simulink model "Inverter_Trifase_PWM_23"  (R2023b)
settings: Solver=ode23s  StartTime=0.0  StopTime=5
values from neighbouring files (symbols this model uses):
  Lc = 10e-3    (= 0.01)    [data.m]
  Rc = 20    [data.m]
  tau = 0.1    [data.m]
  Tc = 100e-6    (= 0.0001)    [data.m]
undefined symbols (not defined in the file or in its folder): DiscIntNeverNeededParam
libraries: fl_lib x80, nesl_utility x51, slpidlib x3, simulink x1
(part 1 of 2)
settings Model: Creator=Student  LastModifiedBy=francesco.bazzani
settings SolverCC: AlgebraicLoopSolver=TrustRegion
settings DataIOCC: SaveFormat=Array  ReturnWorkspaceOutputs=off
settings DebuggingCC: UnconnectedInputMsg=warning  UnconnectedOutputMsg=warning  UnconnectedLineMsg=warning  ArithmeticOperatorsInVariantConditions=warning
settings ModelReferenceCC: EnableRefExpFcnMdlSchedulingChecks=on
settings SFSimCC: SimUseLocalCustomCode=off  CustomCodeUndefinedFunction=UseInterfaceOnly
settings RTWCC: RTWUseLocalCustomCode=off
settings CodeAppCC: StateflowObjectComments=on
settings SimscapeCC: SimscapeNormalizeSystem=off

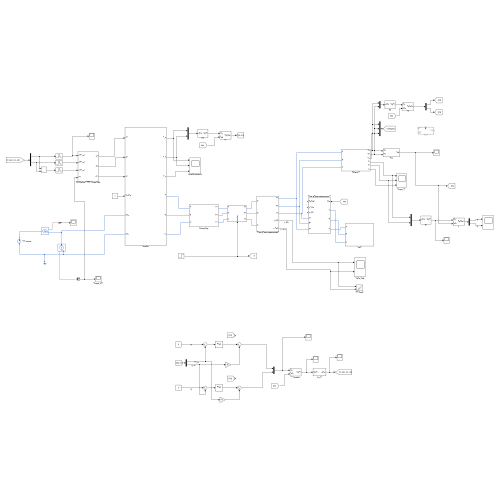
[thumbnail: Simulink's stored preview of the top-level diagram]
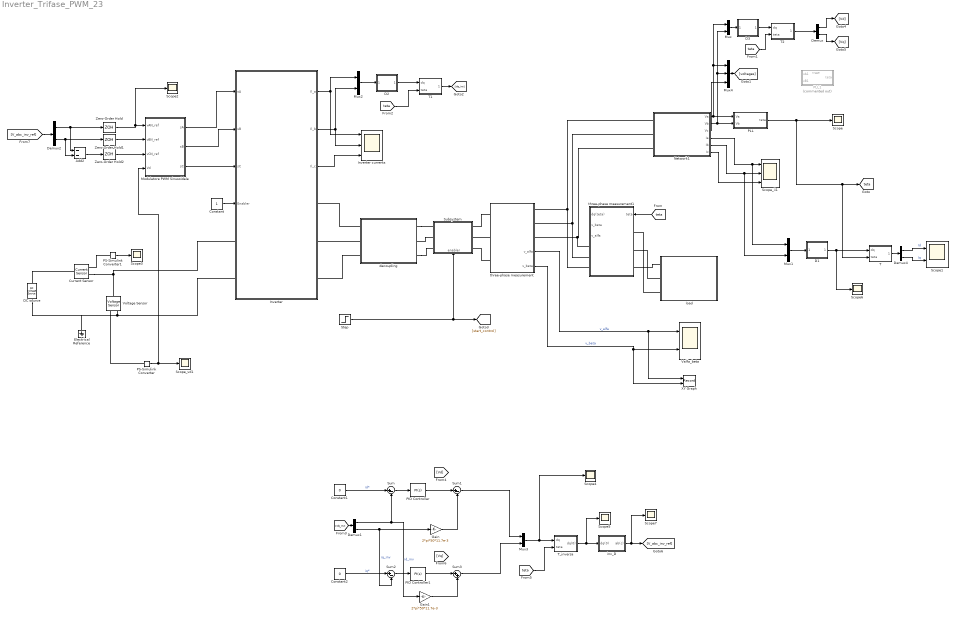
== system Inverter_Trifase_PWM_23 ==
  Add2 : Sum  Inputs=--
  Constant : Constant
  Constant1 : Constant  Value=0
  Constant2 : Constant  Value=0
  Current Sensor : fl_lib/Electrical/Electrical Sensors/Current Sensor
  D1 : Subsystem
  D2 : Subsystem
  D3 : Subsystem
  DC source : fl_lib/Electrical/Electrical Sources/DC Voltage Source  v0=Vd V
  Demux{,1..2,4} (4 alike) : Demux  Outputs=2
  Electrical Reference : fl_lib/Electrical/Electrical Elements/Electrical Reference
  Gain : Gain  Gain=2*pi*50*11.7e-3
  Gain1 : Gain  Gain=2*pi*50*11.7e-3
  Inverter : Subsystem
  Inverter currents : Scope  NumInputPorts=3
  Modulatore PWM Sinusoidale : Subsystem
  Mux{,1..3} (4 alike) : Mux  Inputs=2
  Mux4 : Mux  Inputs=3
  Network1 : Subsystem  mask{E_eff=230, f=50, phi=0}
      mask prompts: f "frequency"; phi "initial_phase"
  PID Controller : slpidlib/PID Controller  Controller=PI  Form=Parallel  TimeDomain=Continuous-time  UseExternalTs=off  SampleTime=-1  IntegratorMethod=Forward Euler  FilterMethod=Forward Euler  ControllerParametersSource=internal  P=Lc/tau  I=Rc/tau  UseKiTs=off  D=0  N=100  UseFilter=on  TunerSelectOption=Transfer Function Based (PID Tuner App)  InitialConditionSource=internal  InitialConditionForIntegrator=0  InitialConditionForFilter=0  DifferentiatorICPrevScaledInput=0  ExternalReset=none  TrackingMode=off  Kt=1  LimitOutput=off  SatLimitsSource=internal  UpperSaturationLimit=inf  LowerSaturationLimit=-inf  LinearizeAsGain=on  AntiWindupMode=none  Kb=1  LimitIntegrator=off  UpperIntegratorSaturationLimit=inf  LowerIntegratorSaturationLimit=-inf  POutMin=[]  POutMax=[]  IOutMin=[]  IOutMax=[]  DOutMin=[]  DOutMax=[]  NOutMin=[]  NOutMax=[]  SumOutMin=[]  SumOutMax=[]  SaturationOutMin=[]  SaturationOutMax=[]  PParamMin=[]  PParamMax=[]  IParamMin=[]  IParamMax=[]  DParamMin=[]  DParamMax=[]  NParamMin=[]  NParamMax=[]  KbParamMin=[]  KbParamMax=[]  KtParamMin=[]  KtParamMax=[]  KbOutMin=[]  KbOutMax=[]  KtOutMin=[]  KtOutMax=[]  IntegratorOutMin=[]  IntegratorOutMax=[]  FilterOutMin=[]  FilterOutMax=[]  SumI1OutMin=[]  SumI1OutMax=[]  SumI2OutMin=[]  SumI2OutMax=[]  SumI3OutMin=[]  SumI3OutMax=[]  SumI4OutMin=[]  SumI4OutMax=[]  SumDOutMin=[]  SumDOutMax=[]  DifferentiatorOutMin=[]  DifferentiatorOutMax=[]  FilterDiffOutCoefMin=[]  FilterDiffOutCoefMax=[]  ReciprocalOutMin=[]  ReciprocalOutMax=[]  SumDenOutMin=[]  SumDenOutMax=[]  SumNumOutMin=[]  SumNumOutMax=[]  DivideOutMin=[]  DivideOutMax=[]  UdiffTsProdOutMin=[]  UdiffTsProdOutMax=[]  NTsProdOutMin=[]  NTsProdOutMax=[]  UintegralTsProdOutMin=[]  UintegralTsProdOutMax=[]  UngainTsProdOutMin=[]  UngainTsProdOutMax=[]  ClampingZeroOutDataTypeStr=Inherit: Inherit via back propagation  ClampingZeroOutMin=[]  ClampingZeroOutMax=[]  FilterDenConstantOutDataTypeStr=Inherit: Inherit via back propagation  FilterDenConstantOutMin=[]  FilterDenConstantOutMax=[]  PCopyOutDataTypeStr=Inherit: Inherit via back propagation  PCopyOutMin=[]  PCopyOutMax=[]  NCopyOutDataTypeStr=Inherit: Inherit via back propagation  NCopyOutMin=[]  NCopyOutMax=[]  IntegratorContinuousStateAttributes=''  IntegratorStateMustResolveToSignalObject=off  IntegratorRTWStateStorageClass=Auto  FilterContinuousStateAttributes=''  FilterStateMustResolveToSignalObject=off  FilterRTWStateStorageClass=Auto  ParallelPVariant=InternalParameters  IdealPVariant=Disabled  IVariant=InternalParameters  DVariant=Disabled  IntegratorVariant=Continuous  SatVariant=Disabled  AWVariant=Passthrough  PCopyVariant=Disabled  TRVariant=Disabled  FdbkBlocksVariant=Forward  IdealPFdbkVariant=Disabled  SatFdbkVariant=Disabled  DerivativeFilterVariant=Disabled  NVariant=Disabled  NCopyVariant=Disabled_SignalSpec  FilterICVariant=Disabled  IntegratorICVariant=InternalICs  ExternalResetVariant=Disabled  TRSumVariant=Passthrough  SumFdbkVariant=Disabled  SumVariant=Sum_PI  TsampFilterVariant=InternalTs  TsampNgainVariant=Passthrough  TsampIntegralVariant=Disabled_SignalSpec  ExternalSaturationOutDataTypeStr=Inherit: Same as second input
  PID Controller1 : slpidlib/PID Controller  Controller=PI  Form=Parallel  TimeDomain=Continuous-time  UseExternalTs=off  SampleTime=-1  IntegratorMethod=Forward Euler  FilterMethod=Forward Euler  ControllerParametersSource=internal  P=Lc/tau  I=Rc/tau  UseKiTs=off  D=0  N=100  UseFilter=on  TunerSelectOption=Transfer Function Based (PID Tuner App)  InitialConditionSource=internal  InitialConditionForIntegrator=0  InitialConditionForFilter=0  DifferentiatorICPrevScaledInput=0  ExternalReset=none  TrackingMode=off  Kt=1  LimitOutput=off  SatLimitsSource=internal  UpperSaturationLimit=inf  LowerSaturationLimit=-inf  LinearizeAsGain=on  AntiWindupMode=none  Kb=1  LimitIntegrator=off  UpperIntegratorSaturationLimit=inf  LowerIntegratorSaturationLimit=-inf  POutMin=[]  POutMax=[]  IOutMin=[]  IOutMax=[]  DOutMin=[]  DOutMax=[]  NOutMin=[]  NOutMax=[]  SumOutMin=[]  SumOutMax=[]  SaturationOutMin=[]  SaturationOutMax=[]  PParamMin=[]  PParamMax=[]  IParamMin=[]  IParamMax=[]  DParamMin=[]  DParamMax=[]  NParamMin=[]  NParamMax=[]  KbParamMin=[]  KbParamMax=[]  KtParamMin=[]  KtParamMax=[]  KbOutMin=[]  KbOutMax=[]  KtOutMin=[]  KtOutMax=[]  IntegratorOutMin=[]  IntegratorOutMax=[]  FilterOutMin=[]  FilterOutMax=[]  SumI1OutMin=[]  SumI1OutMax=[]  SumI2OutMin=[]  SumI2OutMax=[]  SumI3OutMin=[]  SumI3OutMax=[]  SumI4OutMin=[]  SumI4OutMax=[]  SumDOutMin=[]  SumDOutMax=[]  DifferentiatorOutMin=[]  DifferentiatorOutMax=[]  FilterDiffOutCoefMin=[]  FilterDiffOutCoefMax=[]  ReciprocalOutMin=[]  ReciprocalOutMax=[]  SumDenOutMin=[]  SumDenOutMax=[]  SumNumOutMin=[]  SumNumOutMax=[]  DivideOutMin=[]  DivideOutMax=[]  UdiffTsProdOutMin=[]  UdiffTsProdOutMax=[]  NTsProdOutMin=[]  NTsProdOutMax=[]  UintegralTsProdOutMin=[]  UintegralTsProdOutMax=[]  UngainTsProdOutMin=[]  UngainTsProdOutMax=[]  ClampingZeroOutDataTypeStr=Inherit: Inherit via back propagation  ClampingZeroOutMin=[]  ClampingZeroOutMax=[]  FilterDenConstantOutDataTypeStr=Inherit: Inherit via back propagation  FilterDenConstantOutMin=[]  FilterDenConstantOutMax=[]  PCopyOutDataTypeStr=Inherit: Inherit via back propagation  PCopyOutMin=[]  PCopyOutMax=[]  NCopyOutDataTypeStr=Inherit: Inherit via back propagation  NCopyOutMin=[]  NCopyOutMax=[]  IntegratorContinuousStateAttributes=''  IntegratorStateMustResolveToSignalObject=off  IntegratorRTWStateStorageClass=Auto  FilterContinuousStateAttributes=''  FilterStateMustResolveToSignalObject=off  FilterRTWStateStorageClass=Auto  ParallelPVariant=InternalParameters  IdealPVariant=Disabled  IVariant=InternalParameters  DVariant=Disabled  IntegratorVariant=Continuous  SatVariant=Disabled  AWVariant=Passthrough  PCopyVariant=Disabled  TRVariant=Disabled  FdbkBlocksVariant=Forward  IdealPFdbkVariant=Disabled  SatFdbkVariant=Disabled  DerivativeFilterVariant=Disabled  NVariant=Disabled  NCopyVariant=Disabled_SignalSpec  FilterICVariant=Disabled  IntegratorICVariant=InternalICs  ExternalResetVariant=Disabled  TRSumVariant=Passthrough  SumFdbkVariant=Disabled  SumVariant=Sum_PI  TsampFilterVariant=InternalTs  TsampNgainVariant=Passthrough  TsampIntegralVariant=Disabled_SignalSpec  ExternalSaturationOutDataTypeStr=Inherit: Same as second input
  PLL : Subsystem
  PLL1 : Subsystem  Commented=on  mask{ki=500, kp=0.5, f=50}
      mask prompts: f "frequency"
  PS-Simulink Converter : nesl_utility/PS-Simulink Converter  PhysicalDomain=network_engine_domain  SubClassName=ps_output  LeftPortType=input  RightPortType=output  PseudoPeriodic=off  Frequencies=[]  VectorFormat=inherit  Unit=inherit  AffineConversion=off
  PS-Simulink Converter1 : nesl_utility/PS-Simulink Converter  PhysicalDomain=network_engine_domain  SubClassName=ps_output  LeftPortType=input  RightPortType=output  PseudoPeriodic=off  Frequencies=[]  VectorFormat=inherit  Unit=inherit  AffineConversion=off
  Scope{,2..7} (7 alike) : Scope
  Scope1 : Scope  NumInputPorts=2
  Scope_ii1 : Scope  NumInputPorts=3
  Scope_vd1 : Scope
  Step : Step  Time=0  SampleTime=0
  Subsystem : Subsystem
      settings: PortSchema="{\"entries\":[{\"content\":{\"sides\":[{\"content\":{\"connectorIds\":[\"LConn1\",\"LConn2\",\"LConn3\"]},\"type\":\"ConnectorPlacement.EquallySpacedRectSide\",\"uuid\":\"d73297a6-9a93-4c36-8ae1-6d58b261bf06\"},{\"content\":{\"connectorIds\":[\"RConn1\",\"RConn2\",\"RConn3\"],\"side\":\"RIGHT\"},\"type\":\"ConnectorPlacement.EquallySpacedRectSide\",\"uuid\":\"6086bef5-aae9-4392-b869-029ceeb45d41\"},{\"content\":{\"side\":\"TOP\"},\"type\":\"ConnectorPlacement.EquallySpacedRectSide\",\"uuid\":\"d2ebd610-1944-41f8-9294-13f98c946317\"},{\"content\":{\"connectorIds\":[\"In1\"],\"side\":\"BOTTOM\"},\"type\":\"ConnectorPlacement.EquallySpacedRectSide\",\"uuid\":\"967f94e7-9c23-48ce-995b-e38326ca9967\"}]},\"type\":\"ConnectorPlacement.EquallySpacedConnector\",\"uuid\":\"e9d282ac-9c88-4679-adaa-ae858ea7366f\"}],\"packageUris\":[\"http://schema.mathworks.com/mf0/Connector/R2020b\"],\"version\":\"1.0\"}"
  Sum : Sum  Inputs=|+-
  Sum1 : Sum  Inputs=|+-
  Sum2 : Sum  Inputs=|+-
  Sum3 : Sum  Inputs=|++
  T : Subsystem
  T1 : Subsystem
  T2 : Subsystem
  T_inversa : Subsystem
  Valfa_beta : Scope  NumInputPorts=2
  Voltage Sensor : fl_lib/Electrical/Electrical Sensors/Voltage Sensor
  XY Graph : Record  FileSettingsInternal="{\"entries\":[{\"content\":{\"excelSettings\":{\"content\":{},\"type\":\"Streamout.ExcelSettings\"}},\"type\":\"Streamout.FileSettingStorage\",\"uuid\":\"\"}],\"packageUris\":[\"http:\\/\\/schema.mathworks.com\\/mf0\\/streamout_blocks\\/R2020a\"],\"version\":\"1.0\"}"  Layout=[1 1]  SignalsInternal="{\"entries\":[{\"content\":{\"signals\":[{\"content\":{\"blockPath\":[],\"dimensions\":[1],\"domain\":\"\",\"lineColor\":\"#77ac30\",\"lineWidth\":2,\"port\":1,\"signalID\":1,\"signalName\":\"v_alfa\"},\"type\":\"RecordBlkView.Signal\",\"uuid\":\"\"},{\"content\":{\"blockPath\":[],\"dimensions\":[1],\"domain\":\"\",\"lineColor\":\"#4dbeee\",\"lineWidth\":2,\"port\":2,\"signalID\":2,\"signalName\":\"v_beta\"},\"type\":\"RecordBlkView.Signal\",\"uuid\":\"\"}]},\"type\":\"RecordBlkView.InputSignals\",\"uuid\":\"\"}],\"packageUris\":[\"http:\\/\\/schema.mathworks.com\\/mf0\\/streamout_blocks\\/R2020a\"],\"version\":\"1.0\"}"  VisualizationBindings="{\"xyplotplugin\":{\"info\":[{\"series\":[],\"subplotID\":1}]}}"  CompatibilityTag=XY
  Zero-Order Hold : ZeroOrderHold  SampleTime=Tc
  Zero-Order Hold1 : ZeroOrderHold  SampleTime=Tc
  Zero-Order Hold2 : ZeroOrderHold  SampleTime=Tc
  decoupling : Subsystem  mask{Rc=1e-9, Lc=9e-3}
      mask prompts: Rc "Resistor"; Lc "Inductance"
  inv_D : Subsystem
  load : Subsystem  mask{Rc=Rc, Lc=Lc, Cc=0.1e-9}
      mask prompts: Rc "Resistor"; Lc "Inductance"; Cc "Capacitance"
  three-phase measurement : Subsystem
      settings: PortSchema="{\"entries\":[{\"content\":{\"sides\":[{\"content\":{\"connectorIds\":[\"LConn1\",\"LConn2\",\"LConn3\"]},\"type\":\"ConnectorPlacement.EquallySpacedRectSide\",\"uuid\":\"32d21379-5403-4c81-86bb-b48365f60f54\"},{\"content\":{\"connectorIds\":[\"RConn1\",\"RConn2\",\"RConn3\",\"Out1\",\"Out2\"],\"side\":\"RIGHT\"},\"type\":\"ConnectorPlacement.EquallySpacedRectSide\",\"uuid\":\"24ab37a8-a81a-4881-af76-f78c15280390\"},{\"content\":{\"side\":\"TOP\"},\"type\":\"ConnectorPlacement.EquallySpacedRectSide\",\"uuid\":\"2c2ce5b3-2749-4524-8cf7-f3135c13c1a5\"}]},\"type\":\"ConnectorPlacement.EquallySpacedConnector\",\"uuid\":\"48562a3f-ee3b-41f1-a0b2-9ed72f3d9b82\"}],\"packageUris\":[\"http://schema.mathworks.com/mf0/Connector/R2020b\"],\"version\":\"1.0\"}"
  three-phase measurement1 : Subsystem
      settings: PortSchema="{\"entries\":[{\"content\":{\"sides\":[{\"content\":{\"connectorIds\":[\"LConn1\",\"LConn2\",\"LConn3\",\"In1\"]},\"type\":\"ConnectorPlacement.EquallySpacedRectSide\",\"uuid\":\"32d21379-5403-4c81-86bb-b48365f60f54\"},{\"content\":{\"connectorIds\":[\"RConn1\",\"RConn2\",\"RConn3\",\"Out1\",\"Out2\",\"Out3\"],\"side\":\"RIGHT\"},\"type\":\"ConnectorPlacement.EquallySpacedRectSide\",\"uuid\":\"24ab37a8-a81a-4881-af76-f78c15280390\"},{\"content\":{\"side\":\"TOP\"},\"type\":\"ConnectorPlacement.EquallySpacedRectSide\",\"uuid\":\"2c2ce5b3-2749-4524-8cf7-f3135c13c1a5\"}]},\"type\":\"ConnectorPlacement.EquallySpacedConnector\",\"uuid\":\"48562a3f-ee3b-41f1-a0b2-9ed72f3d9b82\"}],\"packageUris\":[\"http://schema.mathworks.com/mf0/Connector/R2020b\"],\"version\":\"1.0\"}"
  tag scope: teta=global
  wires:
  Zero-Order Hold/1 -> Scope2/1, Modulatore PWM Sinusoidale/1(vAN_ref)
  Zero-Order Hold1/1 -> Modulatore PWM Sinusoidale/2(vBN_ref)
  Zero-Order Hold2/1 -> Modulatore PWM Sinusoidale/3(vCN_ref)
  PS-Simulink Converter/1 -> Modulatore PWM Sinusoidale/4(Vd), Scope_vd1/1
  Modulatore PWM Sinusoidale/2(sB) -> Inverter/2(sB)
  Modulatore PWM Sinusoidale/3(sC) -> Inverter/3(sC)
  Modulatore PWM Sinusoidale/1(sA) -> Inverter/1(sA)
  three-phase measurement/1(v_alfa) -> Valfa_beta/1, XY Graph/1  "v_alfa"
  three-phase measurement/2(v_beta) -> XY Graph/2, Valfa_beta/2  "v_beta"
  PLL/1(teta) -> T/2(teta), [teta], Scope/1
  Network1/1(Va) -> Mux/1, Mux4/1, PLL/1(Va)
  Network1/2(Vb) -> Mux/2, Mux4/2, PLL/2(Vb)
  Network1/6(Ic) -> Scope_ii1/3
  Network1/5(Ib) -> Mux1/2, Scope_ii1/2
  Mux1/1 -> D1/1(ab(c))
  Network1/4(Ia) -> Mux1/1, Scope_ii1/1
  PS-Simulink Converter1/1 -> Scope3/1
  Inverter/1(Il_a) -> Inverter currents/1, Mux2/1
  Inverter/2(Il_b) -> Inverter currents/2, Mux2/2
  Inverter/3(Il_c) -> Inverter currents/3
  Mux2/1 -> D2/1(ab(c))
  D2/1(dq(0)) -> T1/1(dq)
  [teta] -> T1/2(teta)
  T1/1(dq(teta)) -> [idq_inv]
  D1/1(dq(0)) -> Scope6/1, T/1(dq)
  T/1(dq(teta)) -> Demux4/1
  Demux4/1 -> Scope1/1  "Id"
  Demux4/2 -> Scope1/2  "Iq"
  Network1/3(Vc) -> Mux4/3
  Mux4/1 -> [voltages]
  Constant/1 -> Inverter/4(Enabler)
  Step/1 -> Subsystem/1(enabler), [start_control]
  [teta] -> three-phase measurement1/1(teta)
  Mux/1 -> D3/1(ab(c))
  D3/1(dq(0)) -> T2/1(dq)
  [teta] -> T2/2(teta)
  T2/1(dq(teta)) -> Demux/1
  Demux/1 -> [Vd]
  Demux/2 -> [Vq]
  Constant1/1 -> Sum/1  "id*"
  [idq_inv] -> Demux1/1
  Demux1/1 -> Gain1/1, Sum/2  "id_inv"
  Sum/1 -> PID Controller/1
  Demux1/2 -> Sum2/2, Gain/1  "iq_inv"
  Gain/1 -> Sum1/2
  PID Controller/1 -> Sum1/1
  PID Controller1/1 -> Sum3/1
  Gain1/1 -> Sum3/2
  Sum2/1 -> PID Controller1/1
  Constant2/1 -> Sum2/1  "iq*"
  Sum1/1 -> Mux3/1
  Sum3/1 -> Mux3/2
  Mux3/1 -> Scope4/1, T_inversa/1(dq)
  [teta] -> T_inversa/2(teta)
  T_inversa/1(dq(0)) -> Scope5/1, inv_D/1(dq(0))
  inv_D/1(ab(c)) -> Scope7/1, [V_abc_inv_ref]
  [V_abc_inv_ref] -> Demux2/1
  Demux2/1 -> Add2/1, Zero-Order Hold/1
  Demux2/2 -> Add2/2, Zero-Order Hold1/1
  Add2/1 -> Zero-Order Hold2/1
  connections:
  Inverter/LConn1 -- Voltage Sensor/LConn1 -- Current Sensor/RConn2
  Voltage Sensor/RConn2 -- DC source/RConn1 -- Electrical Reference/LConn1 -- Inverter/LConn2
  PS-Simulink Converter/LConn1 -- Voltage Sensor/RConn1
  Network1/LConn1 -- three-phase measurement1/RConn1 -- three-phase measurement/RConn1
  Network1/LConn2 -- three-phase measurement1/RConn2 -- three-phase measurement/RConn2
  Network1/LConn3 -- three-phase measurement1/RConn3 -- three-phase measurement/RConn3
  Current Sensor/LConn1 -- DC source/LConn1
  PS-Simulink Converter1/LConn1 -- Current Sensor/RConn1
  three-phase measurement/LConn1 -- Subsystem/LConn1
  three-phase measurement/LConn2 -- Subsystem/LConn2
  three-phase measurement/LConn3 -- Subsystem/LConn3
  decoupling/LConn1 -- Inverter/RConn1
  decoupling/LConn2 -- Inverter/RConn2
  decoupling/LConn3 -- Inverter/RConn3
  Subsystem/RConn2 -- decoupling/RConn2
  decoupling/RConn3 -- Subsystem/RConn3
  decoupling/RConn1 -- Subsystem/RConn1
  load/LConn1 -- three-phase measurement1/LConn1
  load/LConn2 -- three-phase measurement1/LConn2
  load/LConn3 -- three-phase measurement1/LConn3

== system Inverter_Trifase_PWM_23/D1 ==
  ab(c) : Inport
  Gain : Gain  Gain=[1 0; 1/sqrt(3) 2/sqrt(3)]  Multiplication=Matrix(K*u)
  dq(0) : Outport
  wires:
  ab(c)/1 -> Gain/1
  Gain/1 -> dq(0)/1

== system Inverter_Trifase_PWM_23/D2 ==
  ab(c) : Inport
  Gain : Gain  Gain=[1 0; 1/sqrt(3) 2/sqrt(3)]  Multiplication=Matrix(K*u)
  dq(0) : Outport
  wires:
  Gain/1 -> dq(0)/1
  ab(c)/1 -> Gain/1

== system Inverter_Trifase_PWM_23/D3 ==
  ab(c) : Inport
  Gain : Gain  Gain=[1 0; 1/sqrt(3) 2/sqrt(3)]  Multiplication=Matrix(K*u)
  dq(0) : Outport
  wires:
  Gain/1 -> dq(0)/1
  ab(c)/1 -> Gain/1

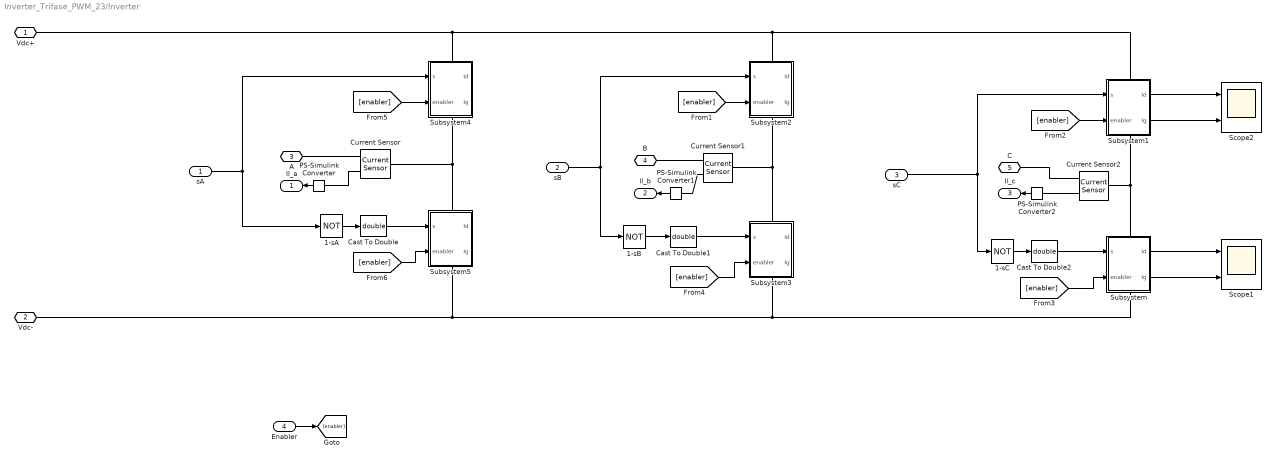
== system Inverter_Trifase_PWM_23/Inverter ==
  sA : Inport
  sB : Inport  Port=2
  sC : Inport  Port=3
  Enabler : Inport  Port=4
  1-sA : Logic  Operator=NOT  AllPortsSameDT=off  OutDataTypeStr=boolean
  1-sB : Logic  Operator=NOT  AllPortsSameDT=off  OutDataTypeStr=boolean
  1-sC : Logic  Operator=NOT  AllPortsSameDT=off  OutDataTypeStr=boolean
  Cast To Double : DataTypeConversion  OutDataTypeStr=double  SaturateOnIntegerOverflow=off  RndMeth=Floor
  Cast To Double1 : DataTypeConversion  OutDataTypeStr=double  SaturateOnIntegerOverflow=off  RndMeth=Floor
  Cast To Double2 : DataTypeConversion  OutDataTypeStr=double  SaturateOnIntegerOverflow=off  RndMeth=Floor
  Current Sensor : fl_lib/Electrical/Electrical Sensors/Current Sensor
  Current Sensor1 : fl_lib/Electrical/Electrical Sensors/Current Sensor
  Current Sensor2 : fl_lib/Electrical/Electrical Sensors/Current Sensor
  PS-Simulink Converter : nesl_utility/PS-Simulink Converter  PhysicalDomain=network_engine_domain  SubClassName=ps_output  LeftPortType=input  RightPortType=output  PseudoPeriodic=off  Frequencies=[]  VectorFormat=inherit  Unit=inherit  AffineConversion=off
  PS-Simulink Converter1 : nesl_utility/PS-Simulink Converter  PhysicalDomain=network_engine_domain  SubClassName=ps_output  LeftPortType=input  RightPortType=output  PseudoPeriodic=off  Frequencies=[]  VectorFormat=inherit  Unit=inherit  AffineConversion=off
  PS-Simulink Converter2 : nesl_utility/PS-Simulink Converter  PhysicalDomain=network_engine_domain  SubClassName=ps_output  LeftPortType=input  RightPortType=output  PseudoPeriodic=off  Frequencies=[]  VectorFormat=inherit  Unit=inherit  AffineConversion=off
  Scope1 : Scope  NumInputPorts=2
  Scope2 : Scope  NumInputPorts=2
  Subsystem : Subsystem
      settings: PortSchema="{\"entries\":[{\"content\":{\"sides\":[{\"content\":{\"connectorIds\":[\"In1\",\"In2\"]},\"type\":\"ConnectorPlacement.EquallySpacedRectSide\",\"uuid\":\"4e5f692d-a64c-483a-ac5e-cd512d23b242\"},{\"content\":{\"connectorIds\":[\"Out1\",\"Out2\"],\"side\":\"RIGHT\"},\"type\":\"ConnectorPlacement.EquallySpacedRectSide\",\"uuid\":\"e12fe3d4-c0cd-4a3e-9242-ad46fbec7d56\"},{\"content\":{\"connectorIds\":[\"LConn1\"],\"side\":\"TOP\"},\"type\":\"ConnectorPlacement.EquallySpacedRectSide\",\"uuid\":\"d4554ec2-8758-4e5e-9cf9-0240d1caee6b\"},{\"content\":{\"connectorIds\":[\"RConn1\"],\"side\":\"BOTTOM\"},\"type\":\"ConnectorPlacement.EquallySpacedRectSide\",\"uuid\":\"09a039c2-054f-4084-afc4-ab4cf2e2d665\"}]},\"type\":\"ConnectorPlacement.EquallySpacedConnector\",\"uuid\":\"56f78543-d3be-4c9c-bdd6-bf2d059f1aee\"}],\"packageUris\":[\"http://schema.mathworks.com/mf0/Connector/R2020b\"],\"version\":\"1.0\"}"
  Subsystem1 : Subsystem
      settings: PortSchema="{\"entries\":[{\"content\":{\"sides\":[{\"content\":{\"connectorIds\":[\"In1\",\"In2\"]},\"type\":\"ConnectorPlacement.EquallySpacedRectSide\",\"uuid\":\"4e5f692d-a64c-483a-ac5e-cd512d23b242\"},{\"content\":{\"connectorIds\":[\"Out1\",\"Out2\"],\"side\":\"RIGHT\"},\"type\":\"ConnectorPlacement.EquallySpacedRectSide\",\"uuid\":\"e12fe3d4-c0cd-4a3e-9242-ad46fbec7d56\"},{\"content\":{\"connectorIds\":[\"LConn1\"],\"side\":\"TOP\"},\"type\":\"ConnectorPlacement.EquallySpacedRectSide\",\"uuid\":\"d4554ec2-8758-4e5e-9cf9-0240d1caee6b\"},{\"content\":{\"connectorIds\":[\"RConn1\"],\"side\":\"BOTTOM\"},\"type\":\"ConnectorPlacement.EquallySpacedRectSide\",\"uuid\":\"09a039c2-054f-4084-afc4-ab4cf2e2d665\"}]},\"type\":\"ConnectorPlacement.EquallySpacedConnector\",\"uuid\":\"56f78543-d3be-4c9c-bdd6-bf2d059f1aee\"}],\"packageUris\":[\"http://schema.mathworks.com/mf0/Connector/R2020b\"],\"version\":\"1.0\"}"
  Subsystem2 : Subsystem
      settings: PortSchema="{\"entries\":[{\"content\":{\"sides\":[{\"content\":{\"connectorIds\":[\"In1\",\"In2\"]},\"type\":\"ConnectorPlacement.EquallySpacedRectSide\",\"uuid\":\"4e5f692d-a64c-483a-ac5e-cd512d23b242\"},{\"content\":{\"connectorIds\":[\"Out1\",\"Out2\"],\"side\":\"RIGHT\"},\"type\":\"ConnectorPlacement.EquallySpacedRectSide\",\"uuid\":\"e12fe3d4-c0cd-4a3e-9242-ad46fbec7d56\"},{\"content\":{\"connectorIds\":[\"LConn1\"],\"side\":\"TOP\"},\"type\":\"ConnectorPlacement.EquallySpacedRectSide\",\"uuid\":\"d4554ec2-8758-4e5e-9cf9-0240d1caee6b\"},{\"content\":{\"connectorIds\":[\"RConn1\"],\"side\":\"BOTTOM\"},\"type\":\"ConnectorPlacement.EquallySpacedRectSide\",\"uuid\":\"09a039c2-054f-4084-afc4-ab4cf2e2d665\"}]},\"type\":\"ConnectorPlacement.EquallySpacedConnector\",\"uuid\":\"56f78543-d3be-4c9c-bdd6-bf2d059f1aee\"}],\"packageUris\":[\"http://schema.mathworks.com/mf0/Connector/R2020b\"],\"version\":\"1.0\"}"
  Subsystem3 : Subsystem
      settings: PortSchema="{\"entries\":[{\"content\":{\"sides\":[{\"content\":{\"connectorIds\":[\"In1\",\"In2\"]},\"type\":\"ConnectorPlacement.EquallySpacedRectSide\",\"uuid\":\"4e5f692d-a64c-483a-ac5e-cd512d23b242\"},{\"content\":{\"connectorIds\":[\"Out1\",\"Out2\"],\"side\":\"RIGHT\"},\"type\":\"ConnectorPlacement.EquallySpacedRectSide\",\"uuid\":\"e12fe3d4-c0cd-4a3e-9242-ad46fbec7d56\"},{\"content\":{\"connectorIds\":[\"LConn1\"],\"side\":\"TOP\"},\"type\":\"ConnectorPlacement.EquallySpacedRectSide\",\"uuid\":\"d4554ec2-8758-4e5e-9cf9-0240d1caee6b\"},{\"content\":{\"connectorIds\":[\"RConn1\"],\"side\":\"BOTTOM\"},\"type\":\"ConnectorPlacement.EquallySpacedRectSide\",\"uuid\":\"09a039c2-054f-4084-afc4-ab4cf2e2d665\"}]},\"type\":\"ConnectorPlacement.EquallySpacedConnector\",\"uuid\":\"56f78543-d3be-4c9c-bdd6-bf2d059f1aee\"}],\"packageUris\":[\"http://schema.mathworks.com/mf0/Connector/R2020b\"],\"version\":\"1.0\"}"
  Subsystem4 : Subsystem
      settings: PortSchema="{\"entries\":[{\"content\":{\"sides\":[{\"content\":{\"connectorIds\":[\"In1\",\"In2\"]},\"type\":\"ConnectorPlacement.EquallySpacedRectSide\",\"uuid\":\"4e5f692d-a64c-483a-ac5e-cd512d23b242\"},{\"content\":{\"connectorIds\":[\"Out1\",\"Out2\"],\"side\":\"RIGHT\"},\"type\":\"ConnectorPlacement.EquallySpacedRectSide\",\"uuid\":\"e12fe3d4-c0cd-4a3e-9242-ad46fbec7d56\"},{\"content\":{\"connectorIds\":[\"LConn1\"],\"side\":\"TOP\"},\"type\":\"ConnectorPlacement.EquallySpacedRectSide\",\"uuid\":\"d4554ec2-8758-4e5e-9cf9-0240d1caee6b\"},{\"content\":{\"connectorIds\":[\"RConn1\"],\"side\":\"BOTTOM\"},\"type\":\"ConnectorPlacement.EquallySpacedRectSide\",\"uuid\":\"09a039c2-054f-4084-afc4-ab4cf2e2d665\"}]},\"type\":\"ConnectorPlacement.EquallySpacedConnector\",\"uuid\":\"56f78543-d3be-4c9c-bdd6-bf2d059f1aee\"}],\"packageUris\":[\"http://schema.mathworks.com/mf0/Connector/R2020b\"],\"version\":\"1.0\"}"
  Subsystem5 : Subsystem
      settings: PortSchema="{\"entries\":[{\"content\":{\"sides\":[{\"content\":{\"connectorIds\":[\"In1\",\"In2\"]},\"type\":\"ConnectorPlacement.EquallySpacedRectSide\",\"uuid\":\"4e5f692d-a64c-483a-ac5e-cd512d23b242\"},{\"content\":{\"connectorIds\":[\"Out1\",\"Out2\"],\"side\":\"RIGHT\"},\"type\":\"ConnectorPlacement.EquallySpacedRectSide\",\"uuid\":\"e12fe3d4-c0cd-4a3e-9242-ad46fbec7d56\"},{\"content\":{\"connectorIds\":[\"LConn1\"],\"side\":\"TOP\"},\"type\":\"ConnectorPlacement.EquallySpacedRectSide\",\"uuid\":\"d4554ec2-8758-4e5e-9cf9-0240d1caee6b\"},{\"content\":{\"connectorIds\":[\"RConn1\"],\"side\":\"BOTTOM\"},\"type\":\"ConnectorPlacement.EquallySpacedRectSide\",\"uuid\":\"09a039c2-054f-4084-afc4-ab4cf2e2d665\"}]},\"type\":\"ConnectorPlacement.EquallySpacedConnector\",\"uuid\":\"56f78543-d3be-4c9c-bdd6-bf2d059f1aee\"}],\"packageUris\":[\"http://schema.mathworks.com/mf0/Connector/R2020b\"],\"version\":\"1.0\"}"
  Vdc+ : PMIOPort  Side=Left
  Vdc- : PMIOPort  Port=2  Side=Left
  A : PMIOPort  Port=3  Side=Right
  B : PMIOPort  Port=4  Side=Right
  C : PMIOPort  Port=5  Side=Right
  Il_a : Outport
  Il_b : Outport  Port=2
  Il_c : Outport  Port=3
  wires:
  1-sA/1 -> Cast To Double/1
  1-sC/1 -> Cast To Double2/1
  1-sB/1 -> Cast To Double1/1
  Cast To Double1/1 -> Subsystem3/1(s)
  Enabler/1 -> [enabler]
  sA/1 -> 1-sA/1, Subsystem4/1(s)
  sB/1 -> 1-sB/1, Subsystem2/1(s)
  sC/1 -> 1-sC/1, Subsystem1/1(s)
  PS-Simulink Converter/1 -> Il_a/1
  PS-Simulink Converter1/1 -> Il_b/1
  PS-Simulink Converter2/1 -> Il_c/1
  Cast To Double2/1 -> Subsystem/1(s)
  [enabler] -> Subsystem/2(enabler)
  [enabler] -> Subsystem1/2(enabler)
  Subsystem1/1(Id) -> Scope2/1
  Subsystem1/2(Ig) -> Scope2/2
  Subsystem/1(Id) -> Scope1/1
  Subsystem/2(Ig) -> Scope1/2
  [enabler] -> Subsystem2/2(enabler)
  [enabler] -> Subsystem3/2(enabler)
  Cast To Double/1 -> Subsystem5/1(s)
  [enabler] -> Subsystem4/2(enabler)
  [enabler] -> Subsystem5/2(enabler)
  connections:
  Subsystem/LConn1 -- Subsystem1/RConn1 -- Current Sensor2/LConn1
  Subsystem1/LConn1 -- Subsystem2/LConn1 -- Vdc+/RConn1 -- Subsystem4/LConn1
  A/RConn1 -- Current Sensor/RConn2
  Current Sensor/RConn1 -- PS-Simulink Converter/LConn1
  Current Sensor1/RConn2 -- B/RConn1
  PS-Simulink Converter1/LConn1 -- Current Sensor1/RConn1
  Current Sensor2/RConn2 -- C/RConn1
  PS-Simulink Converter2/LConn1 -- Current Sensor2/RConn1
  Subsystem3/RConn1 -- Subsystem5/RConn1 -- Vdc-/RConn1 -- Subsystem/RConn1
  Subsystem3/LConn1 -- Current Sensor1/LConn1 -- Subsystem2/RConn1
  Subsystem5/LConn1 -- Current Sensor/LConn1 -- Subsystem4/RConn1

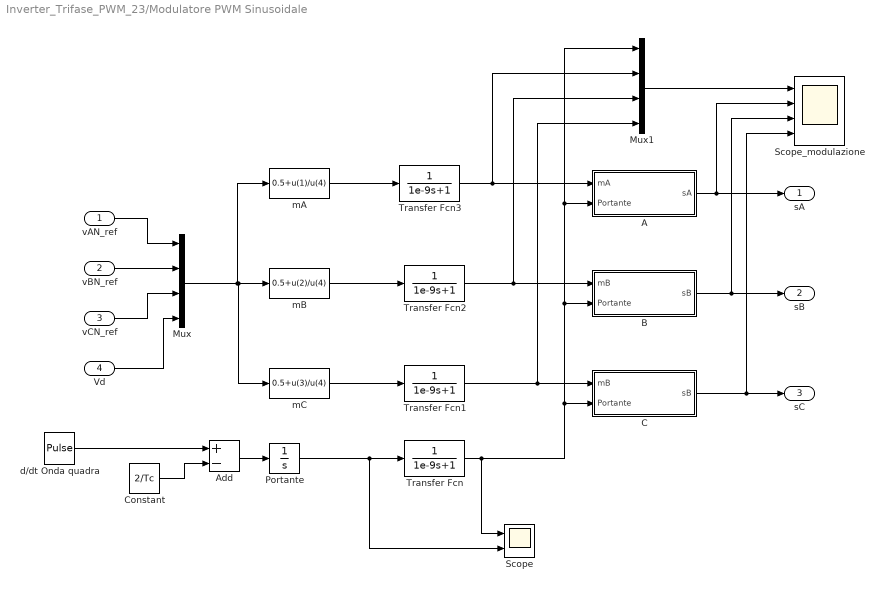
== system Inverter_Trifase_PWM_23/Modulatore PWM Sinusoidale ==
  vAN_ref : Inport
  vBN_ref : Inport  Port=2
  vCN_ref : Inport  Port=3
  Vd : Inport  Port=4
  A : Subsystem
  Add : Sum  Inputs=+-
  B : Subsystem
  C : Subsystem
  Constant : Constant  Value=2/Tc
  Mux : Mux
  Mux1 : Mux
  Portante : Integrator
  Scope : Scope  NumInputPorts=2
  Scope_modulazione : Scope  NumInputPorts=4
  Transfer Fcn{,1..3} (4 alike) : TransferFcn  Denominator=[1e-9 1]
  d/dt Onda quadra : DiscretePulseGenerator  PulseType=Time based  Amplitude=4/Tc  Period=Tc  PulseWidth=50
  mA : Fcn  Expr=0.5+u(1)/u(4)
  mB : Fcn  Expr=0.5+u(2)/u(4)
  mC : Fcn  Expr=0.5+u(3)/u(4)
  sA : Outport  VectorParamsAs1DForOutWhenUnconnected=off
  sB : Outport  Port=2  VectorParamsAs1DForOutWhenUnconnected=off
  sC : Outport  Port=3  VectorParamsAs1DForOutWhenUnconnected=off
  wires:
  d/dt Onda quadra/1 -> Add/1
  Constant/1 -> Add/2
  Add/1 -> Portante/1
  mA/1 -> Transfer Fcn3/1
  Portante/1 -> Scope/2, Transfer Fcn/1
  mB/1 -> Transfer Fcn2/1
  A/1(sA) -> Scope_modulazione/2, sA/1
  B/1(sB) -> Scope_modulazione/3, sB/1
  Mux1/1 -> Scope_modulazione/1
  vAN_ref/1 -> Mux/1
  vBN_ref/1 -> Mux/2
  vCN_ref/1 -> Mux/3
  Vd/1 -> Mux/4
  mC/1 -> Transfer Fcn1/1
  C/1(sB) -> Scope_modulazione/4, sC/1
  Mux/1 -> mA/1, mC/1, mB/1
  Transfer Fcn/1 -> Scope/1, C/2(Portante), B/2(Portante), A/2(Portante), Mux1/1
  Transfer Fcn1/1 -> Mux1/4, C/1(mB)
  Transfer Fcn2/1 -> Mux1/3, B/1(mB)
  Transfer Fcn3/1 -> Mux1/2, A/1(mA)

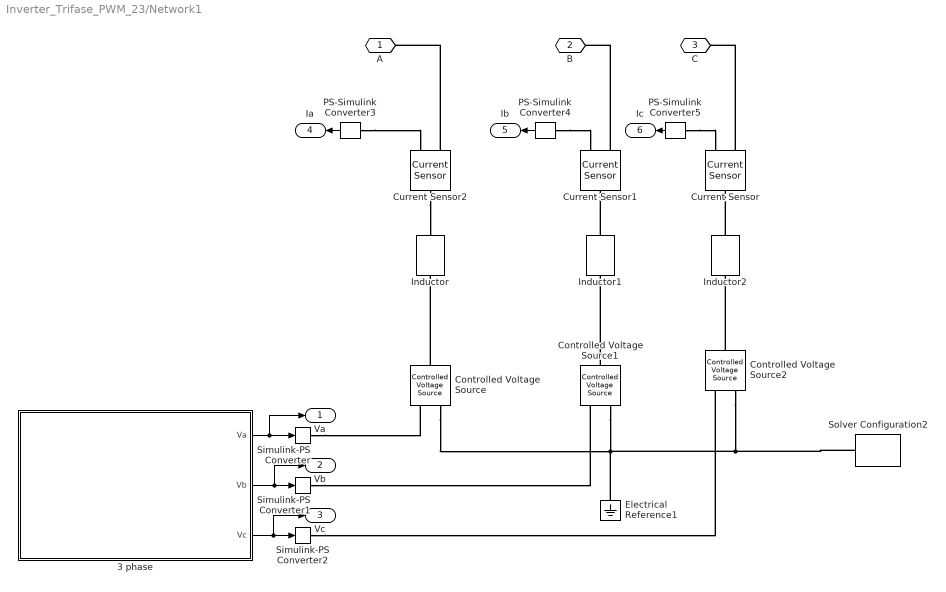
== system Inverter_Trifase_PWM_23/Network1 ==
  3 phase : Subsystem  mask{f=f, Vp=E_eff*sqrt(2)}
      mask prompts: f "Frequency [Hz]"; Vp "Peak value [V]"
  Controlled Voltage Source : fl_lib/Electrical/Electrical Sources/Controlled Voltage Source
  Controlled Voltage Source1 : fl_lib/Electrical/Electrical Sources/Controlled Voltage Source
  Controlled Voltage Source2 : fl_lib/Electrical/Electrical Sources/Controlled Voltage Source
  Current Sensor : fl_lib/Electrical/Electrical Sensors/Current Sensor
  Current Sensor1 : fl_lib/Electrical/Electrical Sensors/Current Sensor
  Current Sensor2 : fl_lib/Electrical/Electrical Sensors/Current Sensor
  Electrical Reference1 : fl_lib/Electrical/Electrical Elements/Electrical Reference
  Inductor : fl_lib/Electrical/Electrical Elements/Inductor  l=2.7e-3 H  r=0 Ohm  g=1e-9 1/Ohm  i_specify=on  i_priority=None  i=0 A  i_nominal_specify=off  i_nominal_value=1  i_nominal_unit=A  v_specify=off  v_priority=None  v=0 V  v_nominal_specify=off  v_nominal_value=1  v_nominal_unit=V  i_L_specify=on  i_L_priority=High  i_L=0 A  i_L_nominal_specify=off  i_L_nominal_value=1  i_L_nominal_unit=A
  Inductor1 : fl_lib/Electrical/Electrical Elements/Inductor  l=2.7e-3 H  r=0 Ohm  g=1e-9 1/Ohm  i_specify=on  i_priority=None  i=0 A  i_nominal_specify=off  i_nominal_value=1  i_nominal_unit=A  v_specify=off  v_priority=None  v=0 V  v_nominal_specify=off  v_nominal_value=1  v_nominal_unit=V  i_L_specify=on  i_L_priority=High  i_L=0 A  i_L_nominal_specify=off  i_L_nominal_value=1  i_L_nominal_unit=A
  Inductor2 : fl_lib/Electrical/Electrical Elements/Inductor  l=2.7e-3 H  r=0 Ohm  g=1e-9 1/Ohm  i_specify=on  i_priority=None  i=0 A  i_nominal_specify=off  i_nominal_value=1  i_nominal_unit=A  v_specify=off  v_priority=None  v=0 V  v_nominal_specify=off  v_nominal_value=1  v_nominal_unit=V  i_L_specify=on  i_L_priority=High  i_L=0 A  i_L_nominal_specify=off  i_L_nominal_value=1  i_L_nominal_unit=A
  PS-Simulink Converter3 : nesl_utility/PS-Simulink Converter  PhysicalDomain=network_engine_domain  SubClassName=ps_output  LeftPortType=input  RightPortType=output  PseudoPeriodic=off  Frequencies=[]  VectorFormat=inherit  Unit=inherit  AffineConversion=off
  PS-Simulink Converter4 : nesl_utility/PS-Simulink Converter  PhysicalDomain=network_engine_domain  SubClassName=ps_output  LeftPortType=input  RightPortType=output  PseudoPeriodic=off  Frequencies=[]  VectorFormat=inherit  Unit=inherit  AffineConversion=off
  PS-Simulink Converter5 : nesl_utility/PS-Simulink Converter  PhysicalDomain=network_engine_domain  SubClassName=ps_output  LeftPortType=input  RightPortType=output  PseudoPeriodic=off  Frequencies=[]  VectorFormat=inherit  Unit=inherit  AffineConversion=off
  Simulink-PS Converter : nesl_utility/Simulink-PS Converter  PhysicalDomain=network_engine_domain  SubClassName=ps_input  LeftPortType=input  RightPortType=output  PseudoPeriodic=off  Frequencies=[]  NoiseDistribution=none  NoiseParameters=[]  Unit=1  AffineConversion=off  FilteringAndDerivatives=provide  SimscapeFilterOrder=1  InputFilterTimeConstant=0.001  UdotUserProvided=0
  Simulink-PS Converter1 : nesl_utility/Simulink-PS Converter  PhysicalDomain=network_engine_domain  SubClassName=ps_input  LeftPortType=input  RightPortType=output  PseudoPeriodic=off  Frequencies=[]  NoiseDistribution=none  NoiseParameters=[]  Unit=1  AffineConversion=off  FilteringAndDerivatives=provide  SimscapeFilterOrder=1  InputFilterTimeConstant=0.001  UdotUserProvided=0
  Simulink-PS Converter2 : nesl_utility/Simulink-PS Converter  PhysicalDomain=network_engine_domain  SubClassName=ps_input  LeftPortType=input  RightPortType=output  PseudoPeriodic=off  Frequencies=[]  NoiseDistribution=none  NoiseParameters=[]  Unit=1  AffineConversion=off  FilteringAndDerivatives=provide  SimscapeFilterOrder=1  InputFilterTimeConstant=0.001  UdotUserProvided=0
  Solver Configuration2 : nesl_utility/Solver Configuration  PhysicalDomain=network_engine_domain  SubClassName=solver  LeftPortType=input  RightPortType=generic  Tones=[]  Harmonics=[]  SimulateNoise=off  Profile=off  UseLocalSampling=off  EnableSwitchedLinearOptims=on  FrequencyDomain=off  UseCCode=off  RelTol=0.001  AbsTol=1e-06  MinStep=1e-09  ToWorkspace=off  RevertToSquareIcSolve=off  NumHomotopyIterations=100  PhasorMode=off  PhasorModeNumHarmonics=1  ConsistencySolver=NEWTON_FTOL  IndexReductionMethod=DerivativeReplacement  DoDC=off  ResidualTolerance=1e-09  ConsistencyTolSource=GLOBAL  ConsistencyAbsTol=0.001  ConsistencyRelTol=0.001  ConsistencyTolFactor=0.001  UseLocalSolver=off  LocalSolverChoice=NE_BACKWARD_EULER_ADVANCER  ResolveIndetEquations=on  FunctionEvalNumThread=1  LocalSolverSampleTime=0.001  DoFixedCost=off  MaxNonlinIter=3  MaxModeIter=2  ComputeImpulses=off  ImpulseIterations=2  LinearAlgebra=Sparse  LinearAlgebraNumThread=0  EquationFormulation=NE_TIME_EF  DelaysMemoryBudget=1024  AutomaticFiltering=on  FilteringTimeConstant=0.001  PartitionStorageMethod=AS_NEEDED  PartitionMemoryBudget=1024  PartitionMethod=ROBUST  MultibodyUseLocalSolver=off  MultibodyLocalSolverChoice=ODE1  MultibodyLocalSolverSampleTime=0.001
  A : PMIOPort  Side=Left
  B : PMIOPort  Port=2  Side=Left
  C : PMIOPort  Port=3  Side=Left
  Va : Outport
  Vb : Outport  Port=2
  Vc : Outport  Port=3
  Ia : Outport  Port=4
  Ib : Outport  Port=5
  Ic : Outport  Port=6
  wires:
  PS-Simulink Converter5/1 -> Ic/1
  PS-Simulink Converter4/1 -> Ib/1
  PS-Simulink Converter3/1 -> Ia/1
  3 phase/2(Vb) -> Vb/1, Simulink-PS Converter1/1
  3 phase/1(Va) -> Va/1, Simulink-PS Converter/1
  3 phase/3(Vc) -> Vc/1, Simulink-PS Converter2/1
  connections:
  PS-Simulink Converter5/LConn1 -- Current Sensor/RConn1
  PS-Simulink Converter4/LConn1 -- Current Sensor1/RConn1
  PS-Simulink Converter3/LConn1 -- Current Sensor2/RConn1
  Current Sensor2/RConn2 -- A/RConn1
  Current Sensor1/RConn2 -- B/RConn1
  Current Sensor/RConn2 -- C/RConn1
  Solver Configuration2/RConn1 -- Controlled Voltage Source/RConn2 -- Electrical Reference1/LConn1 -- Controlled Voltage Source1/RConn2 -- Controlled Voltage Source2/RConn2
  Current Sensor2/LConn1 -- Inductor/LConn1
  Controlled Voltage Source/LConn1 -- Inductor/RConn1
  Inductor1/LConn1 -- Current Sensor1/LConn1
  Inductor2/LConn1 -- Current Sensor/LConn1
  Controlled Voltage Source1/LConn1 -- Inductor1/RConn1
  Controlled Voltage Source2/LConn1 -- Inductor2/RConn1
  Simulink-PS Converter/RConn1 -- Controlled Voltage Source/RConn1
  Simulink-PS Converter1/RConn1 -- Controlled Voltage Source1/RConn1
  Simulink-PS Converter2/RConn1 -- Controlled Voltage Source2/RConn1

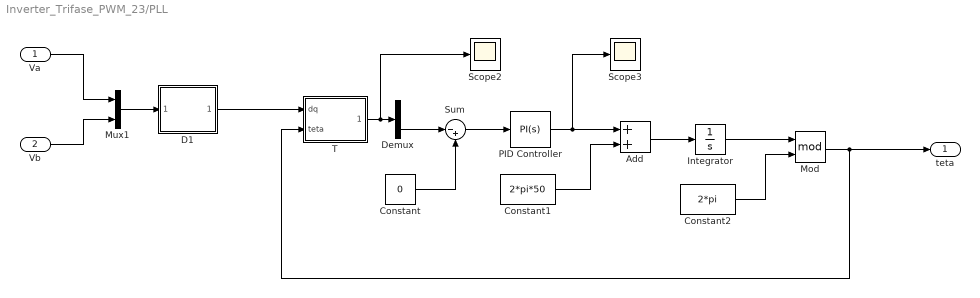
== system Inverter_Trifase_PWM_23/PLL ==
  Va : Inport
  Vb : Inport  Port=2
  Add : Sum
  Constant : Constant  Value=0
  Constant1 : Constant  Value=2*pi*50
  Constant2 : Constant  Value=2*pi
  D1 : Subsystem
  Demux : Demux  Outputs=2
  Integrator : Integrator
  Mod : Math  Operator=mod
  Mux1 : Mux  Inputs=2
  PID Controller : slpidlib/PID Controller  Controller=PI  Form=Parallel  TimeDomain=Continuous-time  UseExternalTs=off  SampleTime=-1  IntegratorMethod=Forward Euler  FilterMethod=Forward Euler  ControllerParametersSource=internal  P=2.7  I=1200  UseKiTs=off  D=0  N=100  UseFilter=on  TunerSelectOption=Transfer Function Based (PID Tuner App)  InitialConditionSource=internal  InitialConditionForIntegrator=0  InitialConditionForFilter=0  DifferentiatorICPrevScaledInput=0  ExternalReset=none  TrackingMode=off  Kt=1  LimitOutput=off  SatLimitsSource=internal  UpperSaturationLimit=inf  LowerSaturationLimit=-inf  LinearizeAsGain=on  AntiWindupMode=none  Kb=1  LimitIntegrator=off  UpperIntegratorSaturationLimit=inf  LowerIntegratorSaturationLimit=-inf  POutMin=[]  POutMax=[]  IOutMin=[]  IOutMax=[]  DOutMin=[]  DOutMax=[]  NOutMin=[]  NOutMax=[]  SumOutMin=[]  SumOutMax=[]  SaturationOutMin=[]  SaturationOutMax=[]  PParamMin=[]  PParamMax=[]  IParamMin=[]  IParamMax=[]  DParamMin=[]  DParamMax=[]  NParamMin=[]  NParamMax=[]  KbParamMin=[]  KbParamMax=[]  KtParamMin=[]  KtParamMax=[]  KbOutMin=[]  KbOutMax=[]  KtOutMin=[]  KtOutMax=[]  IntegratorOutMin=[]  IntegratorOutMax=[]  FilterOutMin=[]  FilterOutMax=[]  SumI1OutMin=[]  SumI1OutMax=[]  SumI2OutMin=[]  SumI2OutMax=[]  SumI3OutMin=[]  SumI3OutMax=[]  SumI4OutMin=[]  SumI4OutMax=[]  SumDOutMin=[]  SumDOutMax=[]  DifferentiatorOutMin=[]  DifferentiatorOutMax=[]  FilterDiffOutCoefMin=[]  FilterDiffOutCoefMax=[]  ReciprocalOutMin=[]  ReciprocalOutMax=[]  SumDenOutMin=[]  SumDenOutMax=[]  SumNumOutMin=[]  SumNumOutMax=[]  DivideOutMin=[]  DivideOutMax=[]  UdiffTsProdOutMin=[]  UdiffTsProdOutMax=[]  NTsProdOutMin=[]  NTsProdOutMax=[]  UintegralTsProdOutMin=[]  UintegralTsProdOutMax=[]  UngainTsProdOutMin=[]  UngainTsProdOutMax=[]  ClampingZeroOutDataTypeStr=Inherit: Inherit via back propagation  ClampingZeroOutMin=[]  ClampingZeroOutMax=[]  FilterDenConstantOutDataTypeStr=Inherit: Inherit via back propagation  FilterDenConstantOutMin=[]  FilterDenConstantOutMax=[]  PCopyOutDataTypeStr=Inherit: Inherit via back propagation  PCopyOutMin=[]  PCopyOutMax=[]  NCopyOutDataTypeStr=Inherit: Inherit via back propagation  NCopyOutMin=[]  NCopyOutMax=[]  IntegratorContinuousStateAttributes=''  IntegratorStateMustResolveToSignalObject=off  IntegratorRTWStateStorageClass=Auto  FilterContinuousStateAttributes=''  FilterStateMustResolveToSignalObject=off  FilterRTWStateStorageClass=Auto  ParallelPVariant=InternalParameters  IdealPVariant=Disabled  IVariant=InternalParameters  DVariant=Disabled  IntegratorVariant=Continuous  SatVariant=Disabled  AWVariant=Passthrough  PCopyVariant=Disabled  TRVariant=Disabled  FdbkBlocksVariant=Forward  IdealPFdbkVariant=Disabled  SatFdbkVariant=Disabled  DerivativeFilterVariant=Disabled  NVariant=Disabled  NCopyVariant=Disabled_SignalSpec  FilterICVariant=Disabled  IntegratorICVariant=InternalICs  ExternalResetVariant=Disabled  TRSumVariant=Passthrough  SumFdbkVariant=Disabled  SumVariant=Sum_PI  TsampFilterVariant=InternalTs  TsampNgainVariant=Passthrough  TsampIntegralVariant=Disabled_SignalSpec  ExternalSaturationOutDataTypeStr=Inherit: Same as second input
  Scope2 : Scope
  Scope3 : Scope
  Sum : Sum  Inputs=|-+
  T : Subsystem
  teta : Outport
  wires:
  Vb/1 -> Mux1/2
  Add/1 -> Integrator/1
  Integrator/1 -> Mod/1
  Constant2/1 -> Mod/2
  Constant/1 -> Sum/2
  Va/1 -> Mux1/1
  Constant1/1 -> Add/2
  Sum/1 -> PID Controller/1
  Mux1/1 -> D1/1(ab(c))
  Mod/1 -> teta/1, T/2(teta)
  T/1(dq(teta)) -> Scope2/1, Demux/1
  D1/1(dq(0)) -> T/1(dq)
  PID Controller/1 -> Scope3/1, Add/1
  Demux/2 -> Sum/1

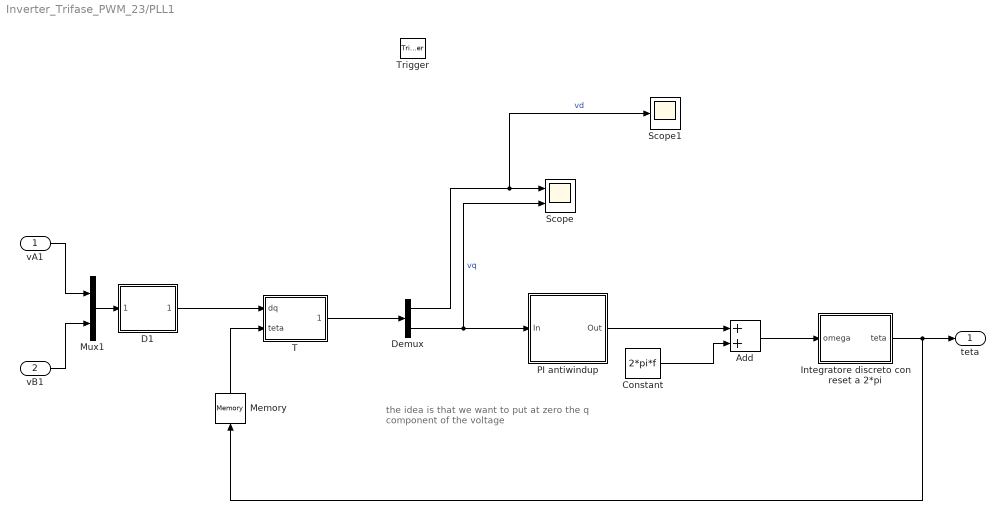
== system Inverter_Trifase_PWM_23/PLL1 ==
  note: the idea is that we want to put at zero the q component of the voltage
  vA1 : Inport
  vB1 : Inport  Port=2
  Trigger : TriggerPort  VariantControl=Variant
  Add : Sum
  Constant : Constant  Value=2*pi*f
  D1 : Subsystem
  Demux : Demux  Outputs=2
  Integratore discreto con reset a 2*pi : Subsystem
  Memory : Memory  InheritSampleTime=on
  Mux1 : Mux  Inputs=2
  PI antiwindup : Subsystem  mask{kp_PLL_edit=kp, ki_PLL_edit=ki, min_PLL=-1000, max_PLL=1000}
      mask prompts: kp_PLL_edit "kp"; ki_PLL_edit "ki"; min_PLL "min PLL"; max_PLL "max PLL"
  Scope : Scope  NumInputPorts=2
  Scope1 : Scope
  T : Subsystem
  teta : Outport
  wires:
  D1/1(dq(0)) -> T/1(dq)
  Mux1/1 -> D1/1(ab(c))
  vB1/1 -> Mux1/2
  vA1/1 -> Mux1/1
  T/1(dq(teta)) -> Demux/1
  Demux/2 -> Scope/2, PI antiwindup/1(In)  "vq"
  Integratore discreto con reset a 2*pi/1(teta) -> Memory/1, teta/1
  Add/1 -> Integratore discreto con reset a 2*pi/1(omega)
  Constant/1 -> Add/2
  PI antiwindup/1(Out) -> Add/1
  Memory/1 -> T/2(teta)
  Demux/1 -> Scope1/1, Scope/1  "vd"

== system Inverter_Trifase_PWM_23/Subsystem ==
  enabler : Inport
  Simulink-PS Converter : nesl_utility/Simulink-PS Converter  PhysicalDomain=network_engine_domain  SubClassName=ps_input  LeftPortType=input  RightPortType=output  PseudoPeriodic=off  Frequencies=[]  NoiseDistribution=none  NoiseParameters=[]  Unit=1  AffineConversion=off  FilteringAndDerivatives=provide  SimscapeFilterOrder=1  InputFilterTimeConstant=0.001  UdotUserProvided=0
  Simulink-PS Converter1 : nesl_utility/Simulink-PS Converter  PhysicalDomain=network_engine_domain  SubClassName=ps_input  LeftPortType=input  RightPortType=output  PseudoPeriodic=off  Frequencies=[]  NoiseDistribution=none  NoiseParameters=[]  Unit=1  AffineConversion=off  FilteringAndDerivatives=provide  SimscapeFilterOrder=1  InputFilterTimeConstant=0.001  UdotUserProvided=0
  Simulink-PS Converter2 : nesl_utility/Simulink-PS Converter  PhysicalDomain=network_engine_domain  SubClassName=ps_input  LeftPortType=input  RightPortType=output  PseudoPeriodic=off  Frequencies=[]  NoiseDistribution=none  NoiseParameters=[]  Unit=1  AffineConversion=off  FilteringAndDerivatives=provide  SimscapeFilterOrder=1  InputFilterTimeConstant=0.001  UdotUserProvided=0
  Switch : fl_lib/Electrical/Electrical Elements/Switch  R_closed=0.01 Ohm  G_open=1e-8 1/Ohm  Threshold=0.5  i_specify=off  i_priority=None  i=0 A  i_nominal_specify=off  i_nominal_value=1  i_nominal_unit=A  v_specify=off  v_priority=None  v=0 V  v_nominal_specify=off  v_nominal_value=1  v_nominal_unit=V
  Switch1 : fl_lib/Electrical/Electrical Elements/Switch  R_closed=0.01 Ohm  G_open=1e-8 1/Ohm  Threshold=0.5  i_specify=off  i_priority=None  i=0 A  i_nominal_specify=off  i_nominal_value=1  i_nominal_unit=A  v_specify=off  v_priority=None  v=0 V  v_nominal_specify=off  v_nominal_value=1  v_nominal_unit=V
  Switch2 : fl_lib/Electrical/Electrical Elements/Switch  R_closed=0.01 Ohm  G_open=1e-8 1/Ohm  Threshold=0.5  i_specify=off  i_priority=None  i=0 A  i_nominal_specify=off  i_nominal_value=1  i_nominal_unit=A  v_specify=off  v_priority=None  v=0 V  v_nominal_specify=off  v_nominal_value=1  v_nominal_unit=V
  A1 : PMIOPort  Side=Left
  B1 : PMIOPort  Port=2  Side=Left
  C1 : PMIOPort  Port=3  Side=Left
  A : PMIOPort  Port=4  Side=Right
  B : PMIOPort  Port=5  Side=Right
  C : PMIOPort  Port=6  Side=Right
  wires:
  enabler/1 -> Simulink-PS Converter1/1, Simulink-PS Converter2/1, Simulink-PS Converter/1
  connections:
  Switch1/LConn1 -- B1/RConn1
  Switch2/LConn1 -- C1/RConn1
  Simulink-PS Converter/RConn1 -- Switch/RConn1
  Switch2/RConn2 -- C/RConn1
  Switch/LConn1 -- A1/RConn1
  Simulink-PS Converter2/RConn1 -- Switch2/RConn1
  Switch/RConn2 -- A/RConn1
  Switch1/RConn2 -- B/RConn1
  Simulink-PS Converter1/RConn1 -- Switch1/RConn1

== system Inverter_Trifase_PWM_23/T ==
  dq : Inport
  teta : Inport  Port=2
  Demux : Demux  Outputs=2
  Fcn : Fcn  Expr=cos(u[3])*u[1]+sin(u[3])*u[2]
  Fcn1 : Fcn  Expr=-sin(u[3])*u[1]+cos(u[3])*u[2]
  Mux : Mux  Inputs=3
  Mux1 : Mux  Inputs=2
  dq(teta) : Outport
  wires:
  Mux1/1 -> dq(teta)/1
  Fcn1/1 -> Mux1/2
  Fcn/1 -> Mux1/1
  Mux/1 -> Fcn/1, Fcn1/1
  teta/1 -> Mux/3
  Demux/2 -> Mux/2
  Demux/1 -> Mux/1
  dq/1 -> Demux/1

== system Inverter_Trifase_PWM_23/T1 ==
  dq : Inport
  teta : Inport  Port=2
  Demux : Demux  Outputs=2
  Fcn : Fcn  Expr=cos(u[3])*u[1]+sin(u[3])*u[2]
  Fcn1 : Fcn  Expr=-sin(u[3])*u[1]+cos(u[3])*u[2]
  Mux : Mux  Inputs=3
  Mux1 : Mux  Inputs=2
  dq(teta) : Outport
  wires:
  dq/1 -> Demux/1
  Demux/1 -> Mux/1
  Demux/2 -> Mux/2
  teta/1 -> Mux/3
  Mux/1 -> Fcn1/1, Fcn/1
  Fcn/1 -> Mux1/1
  Fcn1/1 -> Mux1/2
  Mux1/1 -> dq(teta)/1

== system Inverter_Trifase_PWM_23/T2 ==
  dq : Inport
  teta : Inport  Port=2
  Demux : Demux  Outputs=2
  Fcn : Fcn  Expr=cos(u[3])*u[1]+sin(u[3])*u[2]
  Fcn1 : Fcn  Expr=-sin(u[3])*u[1]+cos(u[3])*u[2]
  Mux : Mux  Inputs=3
  Mux1 : Mux  Inputs=2
  dq(teta) : Outport
  wires:
  Mux1/1 -> dq(teta)/1
  Fcn1/1 -> Mux1/2
  Fcn/1 -> Mux1/1
  Mux/1 -> Fcn/1, Fcn1/1
  teta/1 -> Mux/3
  Demux/2 -> Mux/2
  Demux/1 -> Mux/1
  dq/1 -> Demux/1

== system Inverter_Trifase_PWM_23/T_inversa ==
  dq : Inport
  teta : Inport  Port=2
  Demux : Demux  Outputs=2
  Fcn : Fcn  Expr=cos(u[3])*u[1]+sin(u[3])*u[2]
  Fcn1 : Fcn  Expr=-sin(u[3])*u[1]+cos(u[3])*u[2]
  Gain8 : Gain  Gain=-1
  Mux : Mux  Inputs=3
  Mux1 : Mux  Inputs=2
  dq(0) : Outport
  wires:
  dq/1 -> Demux/1
  Demux/1 -> Mux/1
  Demux/2 -> Mux/2
  Mux/1 -> Fcn/1, Fcn1/1
  Fcn/1 -> Mux1/1
  Fcn1/1 -> Mux1/2
  Mux1/1 -> dq(0)/1
  teta/1 -> Gain8/1
  Gain8/1 -> Mux/3

== system Inverter_Trifase_PWM_23/decoupling ==
  Inductor : fl_lib/Electrical/Electrical Elements/Inductor  l=Lc H  r=0 Ohm  g=1e-9 1/Ohm  i_specify=on  i_priority=None  i=0 A  i_nominal_specify=off  i_nominal_value=1  i_nominal_unit=A  v_specify=off  v_priority=None  v=0 V  v_nominal_specify=off  v_nominal_value=1  v_nominal_unit=V  i_L_specify=off  i_L_priority=High  i_L=0 A  i_L_nominal_specify=off  i_L_nominal_value=1  i_L_nominal_unit=A
  Inductor1 : fl_lib/Electrical/Electrical Elements/Inductor  l=Lc H  r=0 Ohm  g=1e-9 1/Ohm  i_specify=on  i_priority=None  i=0 A  i_nominal_specify=off  i_nominal_value=1  i_nominal_unit=A  v_specify=off  v_priority=None  v=0 V  v_nominal_specify=off  v_nominal_value=1  v_nominal_unit=V  i_L_specify=off  i_L_priority=High  i_L=0 A  i_L_nominal_specify=off  i_L_nominal_value=1  i_L_nominal_unit=A
  Inductor2 : fl_lib/Electrical/Electrical Elements/Inductor  l=Lc H  r=0 Ohm  g=1e-9 1/Ohm  i_specify=on  i_priority=None  i=0 A  i_nominal_specify=off  i_nominal_value=1  i_nominal_unit=A  v_specify=off  v_priority=None  v=0 V  v_nominal_specify=off  v_nominal_value=1  v_nominal_unit=V  i_L_specify=off  i_L_priority=High  i_L=0 A  i_L_nominal_specify=off  i_L_nominal_value=1  i_L_nominal_unit=A
  Resistor : fl_lib/Electrical/Electrical Elements/Resistor  R=Rc Ohm  i_specify=on  i_priority=None  i=0 A  i_nominal_specify=off  i_nominal_value=1  i_nominal_unit=A  v_specify=off  v_priority=None  v=0 V  v_nominal_specify=off  v_nominal_value=1  v_nominal_unit=V
  Resistor1 : fl_lib/Electrical/Electrical Elements/Resistor  R=Rc Ohm  i_specify=on  i_priority=None  i=0 A  i_nominal_specify=off  i_nominal_value=1  i_nominal_unit=A  v_specify=off  v_priority=None  v=0 V  v_nominal_specify=off  v_nominal_value=1  v_nominal_unit=V
  Resistor2 : fl_lib/Electrical/Electrical Elements/Resistor  R=Rc Ohm  i_specify=on  i_priority=None  i=0 A  i_nominal_specify=off  i_nominal_value=1  i_nominal_unit=A  v_specify=off  v_priority=None  v=0 V  v_nominal_specify=off  v_nominal_value=1  v_nominal_unit=V
  A : PMIOPort  Side=Left
  B : PMIOPort  Port=2  Side=Left
  C : PMIOPort  Port=3  Side=Left
  A1 : PMIOPort  Port=4  Side=Right
  B1 : PMIOPort  Port=5  Side=Right
  C1 : PMIOPort  Port=6  Side=Right
  connections:
  Inductor2/LConn1 -- Resistor2/RConn1
  Inductor1/LConn1 -- Resistor1/RConn1
  Resistor1/LConn1 -- B/RConn1
  Inductor/LConn1 -- Resistor/RConn1
  Resistor2/LConn1 -- C/RConn1
  Resistor/LConn1 -- A/RConn1
  A1/RConn1 -- Inductor/RConn1
  B1/RConn1 -- Inductor1/RConn1
  C1/RConn1 -- Inductor2/RConn1

== system Inverter_Trifase_PWM_23/inv_D ==
  dq(0) : Inport
  Gain : Gain  Gain=[1 0; -1/2 sqrt(3)/2]  Multiplication=Matrix(K*u)
  ab(c) : Outport
  wires:
  Gain/1 -> ab(c)/1
  dq(0)/1 -> Gain/1
